simulink model "PSInput_Experiment"  (R2025a)
settings: Solver=VariableStepAuto  StartTime=0.0  StopTime=10.0  RelTol=1e-3
undefined symbols (not defined in the file or in its folder): c1, c2
libraries: fl_lib x4
settings Model: Creator=isaacito  LastModifiedBy=isaacito

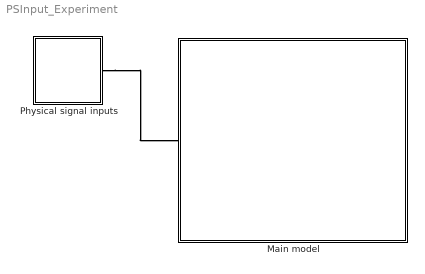
== system PSInput_Experiment ==
  Main model : Subsystem
  Physical signal inputs : Subsystem
  connections:
  Physical signal inputs/RConn1 -- Main model/LConn1

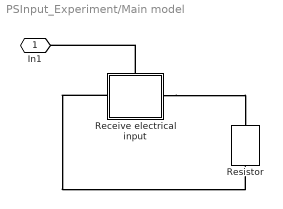
== system PSInput_Experiment/Main model ==
  Receive electrical input : Subsystem
      settings: PortSchema="{\"entries\":[{\"content\":{\"sides\":[{\"content\":{},\"type\":\"ConnectorPlacement.EquallySpacedRectSide\",\"uuid\":\"1f18aba0-f0f2-4650-8d1d-72a31ca39181\"},{\"content\":{\"connectorIds\":[\"RConn1\"],\"side\":\"RIGHT\"},\"type\":\"ConnectorPlacement.EquallySpacedRectSide\",\"uuid\":\"864b9971-1efb-4e52-b635-0618542df393\"},{\"content\":{\"connectorIds\":[\"LConn1\"],\"side\":\"TOP\"},\"type\":\"ConnectorPlacement.EquallySpacedRectSide\",\"uuid\":\"59a8b60d-e212-48a2-b18d-e8d9828a47db\"},{\"content\":{\"connectorIds\":[\"RConn2\"],\"side\":\"BOTTOM\"},\"type\":\"ConnectorPlacement.EquallySpacedRectSide\",\"uuid\":\"48fdcc00-7e89-40fe-a9d7-1dd8a172ba98\"}]},\"type\":\"ConnectorPlacement.EquallySpacedConnector\",\"uuid\":\"08312f7d-61e5-41d3-b4a2-9499a77f24d2\"}],\"packageUris\":[\"http://schema.mathworks.com/mf0/Connector/R2020b\"],\"version\":\"1.0\"}"
  Resistor : fl_lib/Electrical/Electrical Elements/Resistor  R=1 Ohm  i_specify=off  i_priority=None  i=0 A  i_nominal_specify=off  i_nominal_value=1  i_nominal_unit=A  v_specify=off  v_priority=None  v=0 V  v_nominal_specify=off  v_nominal_value=1  v_nominal_unit=V
  In1 : PMIOPort  Side=Left
  connections:
  Receive electrical input/RConn1 -- In1/RConn1
  Receive electrical input/LConn1 -- Resistor/LConn1
  Receive electrical input/RConn2 -- Resistor/RConn1

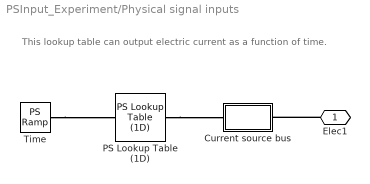
== system PSInput_Experiment/Physical signal inputs ==
  note: This lookup table can output electric current as a function of time.
  Current source bus : Subsystem
  PS Lookup Table (1D) : fl_lib/Physical Signals/Lookup Tables/PS Lookup Table (1D)  x=[1, 2, 3, 4, 5]  f=[0, 1, 2, 3, 4]  interp_method=simscape.enum.interpolation.linear  extrap_method=simscape.enum.extrapolation.linear
  Time : fl_lib/Physical Signals/Sources/PS Ramp  slope=1 1/s  start_time=0 s  initial_output=0  ZeroCross=false
  Elec1 : PMIOPort  Side=Right
  connections:
  Time/RConn1 -- PS Lookup Table (1D)/LConn1
  Elec1/RConn1 -- Current source bus/RConn1
  PS Lookup Table (1D)/RConn1 -- Current source bus/LConn1

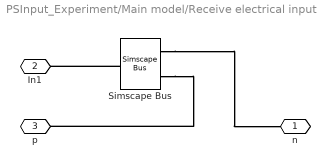
== system PSInput_Experiment/Main model/Receive electrical input ==
  Simscape Bus : SimscapeBus  HierarchyStrings=c1;c2
  n : PMIOPort  Side=Left
  In1 : PMIOPort  Port=2  Side=Right
  p : PMIOPort  Port=3  Side=Right
  connections:
  Simscape Bus/LConn2 -- p/RConn1
  Simscape Bus/RConn1 -- In1/RConn1
  Simscape Bus/LConn1 -- n/RConn1

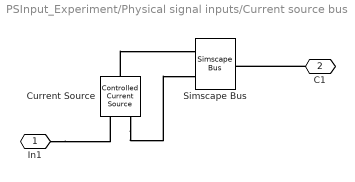
== system PSInput_Experiment/Physical signal inputs/Current source bus ==
  Current Source : fl_lib/Electrical/Electrical Sources/Controlled Current Source
  Simscape Bus : SimscapeBus  HierarchyStrings=c1;c2
  In1 : PMIOPort  Side=Left
  C1 : PMIOPort  Port=2  Side=Right
  connections:
  Current Source/RConn2 -- Simscape Bus/LConn2
  In1/RConn1 -- Current Source/RConn1
  Current Source/LConn1 -- Simscape Bus/LConn1
  C1/RConn1 -- Simscape Bus/RConn1
